simulink model "DAS"  (R2012b)
settings: Solver=FixedStepDiscrete  StartTime=0.0  StopTime=inf  FixedStep=0.1  RelTol=1e-3
PreLoadFcn:
  | if exist('tl_preloadfcn','file'), tl_preloadfcn(gcs,101); end
PostLoadFcn:
  | if exist('tl_postloadfcn','file'), tl_postloadfcn(gcs,101); end
InitFcn:
  | if exist('tlds_init','file'), tlds_init(gcs); end
StartFcn:
  | if exist('tlds_start','file'), tlds_start(gcs); end
StopFcn:
  | if exist('tlds_stop','file'), tlds_stop(gcs); end
undefined symbols (not defined in the file): A, B, C, Dd, DEMO_FAS_Accusti_Threshold_Time, DEMO_FAS_BrakeBooster_Threshold, DEMO_FAS_CC_DELTA, DEMO_FAS_CC_Lvl2_Round, DEMO_FAS_CC_Min_Value, DEMO_FAS_Distance_Treshold_Far, DEMO_FAS_Distance_Treshold_Med, DEMO_FAS_Distance_Treshold_Near, DEMO_FAS_Distronic, DEMO_FAS_Emerg_Brake_Force1, DEMO_FAS_Emerg_Brake_Force2, DEMO_FAS_Emerg_Brake_Time1, DEMO_FAS_Emerg_Brake_Time2, DEMO_FAS_EmergencyBrake, DEMO_FAS_FollowToStop, DEMO_FAS_Limiter, DEMO_FAS_Limiter_DELTA, DEMO_FAS_Neg_Max_ms, DEMO_FAS_Opti_Threshold_Time, DEMO_FAS_Repeater, DEMO_FAS_Repeater_Time, DEMO_FAS_Signdetection, DEMO_FAS_Tempomat
(part 8 of 11)

== system DAS/DEMO_FAS/DEMO_FAS/Subsystem/DEMO_FAS/DEMO_FAS_Funktion/Tempomat/Tempomat_Function/CC_Enabled/Tempomat_Active ==
  V_Vehicle_kmh : Inport
  Action Port : ActionPort  ActionType=then
  Data Store Read1 : DataStoreRead  Description=|  DataStoreName=DEMO_FAS_V_CCSetValue  mask(TL_DataStoreRead){data={'logdata',{'plotchannels',[]},'date',735342.58789737266}}
      | Data Store Read block of dSPACE TargetLink.
      | Use this block to specify inputs from global variables within the production code application.
      settings: DeleteFcn=if exist('delete_tlblock','file')==2,delete_tlblock(gcbh);end  NameChangeFcn=if exist('rename_tlblock','file')==2,rename_tlblock(gcbh);end  OpenFcn=if exist('tl_open_blockdlg','file')==2,tl_open_blockdlg(gcbh);else,open_system(gcbh,'parameter');end
      mask Help: eval(['if exist(''tl_online_help'',''file'') == 2, tl_online_help(''Topic'',''TL_DataStoreRead''),else, web([''jar:file:///'',matlabroot,''/help/toolbox/simulink/help.jar!/slref/' lower(get_param(gcbh,'Blocktype')) '.html''], ''-helpbrowser''),end'])
      mask Display: plot([-0.05, 1.05, NaN, -0.05, 1.05],[.01, .01, NaN, .99, .99])
  Sum : Sum  Description=|  Inputs=-+  mask(TL_Sum){data={'logdata',{'plotchannels',[]},'date',735350.38399912033}}
      | Sum block of dSPACE TargetLink.
      | 
      | Output signal is equal to the sum of the input signals.
      | The list of signs is specified according to conventions for Simulink Sum blocks.
      settings: CopyFcn=if exist('tl_reset_reviewflag') == 2, tl_reset_reviewflag(gcbh); end  DeleteFcn=if exist('delete_tlblock','file')==2,delete_tlblock(gcbh);end  NameChangeFcn=if exist('rename_tlblock','file')==2,rename_tlblock(gcbh);end  OpenFcn=if exist('tl_open_blockdlg','file')==2,tl_open_blockdlg(gcbh);else,open_system(gcbh,'parameter');end
      mask Help: eval(['if exist(''tl_online_help'',''file'') == 2, tl_online_help(''Topic'',''TL_Sum''),else, web([''jar:file:///'',matlabroot,''/help/toolbox/simulink/help.jar!/slref/' lower(get_param(gcbh,'Blocktype')) '.html''], ''-helpbrowser''),end'])
      mask Display: plot([-0.05, 1.05, NaN, -0.05, 1.05],[.01, .01, NaN, .99, .99])
  VERSION_INFO : Subsystem  mask(VERSION_INFO_BLOCK){versinfo_data=struct('modname','DEMO_FAS/DEMO_FAS_Funktion/Tempomat/Tempomat_Function/CC_Enabled/Tempomat_Active','version','1.1.1','date','18-Apr-2013','author','YVEDUHR','modtype',3,'variant',0,'remark',{{'~'}},'copyright',['Daimler AG'],'SGMLdescr','','prefix','','pfx_act',0,'ntselect',3,'asize',0), versinfo_string=Model: DEMO_FAS/DEMO_FAS_Funktion/Tempomat/Tempomat_Function/CC_Enabled/Tempomat_Active\nVersion: 1.1.1\nDate: 18-Apr-2013\nAuthor: YVEDUHR\nModule: INTERNAL\n\nAll copyrights by Daimler AG}
      mask prompts: versinfo_data "Mask Parameter 1"; versinfo_string "Mask Parameter 2"
      mask help:
      | This is a Version Info Subsystem (empty)
      | All version Information is stored in Parameter "versinfo_data" and displayed
      settings: OpenFcn=edit_subsys_info('init')
      mask Display: disp(versinfo_string);
  V_CC_delta_kmh : Outport  InitialOutput=0
  wires:
  V_Vehicle_kmh/1 -> Sum/1
  Sum/1 -> V_CC_delta_kmh/1  "V_CC_delta_kmh"
  Data Store Read1/1 -> Sum/2

== system DAS/DEMO_FAS/DEMO_FAS/Subsystem/DEMO_FAS/DEMO_FAS_Funktion/Tempomat/Tempomat_Function/CC_Enabled/Tempomat_Deactive ==
  Action Port : ActionPort  ActionType=else
  Constant : Constant  Value=0  mask(TL_Constant){data={'date',735339.6780933796}}
      settings: CopyFcn=if exist('tl_reset_reviewflag') == 2, tl_reset_reviewflag(gcbh); end  DeleteFcn=if exist('delete_tlblock','file')==2,delete_tlblock(gcbh);end  NameChangeFcn=if exist('rename_tlblock','file')==2,rename_tlblock(gcbh);end  OpenFcn=if exist('tl_open_blockdlg','file')==2,tl_open_blockdlg(gcbh);else,open_system(gcbh,'parameter');end
      mask Help: eval(['if exist(''tl_online_help'',''file'') == 2, tl_online_help(''Topic'',''TL_Constant''),else, web([''jar:file:///'',matlabroot,''/help/toolbox/simulink/help.jar!/slref/' lower(get_param(gcbh,'Blocktype')) '.html''], ''-helpbrowser''),end'])
      mask Display: plot([-0.05, 1.05, NaN, -0.05, 1.05],[.01, .01, NaN, .99, .99])
  VERSION_INFO : Subsystem  mask(VERSION_INFO_BLOCK){versinfo_data=struct('modname','DEMO_FAS/DEMO_FAS_Funktion/Tempomat/Tempomat_Function/CC_Enabled/Tempomat_Deactive','version','1.1.1','date','18-Apr-2013','author','YVEDUHR','modtype',3,'variant',0,'remark',{{'~'}},'copyright',['Daimler AG'],'SGMLdescr','','prefix','','pfx_act',0,'ntselect',3,'asize',0), versinfo_string=Model: DEMO_FAS/DEMO_FAS_Funktion/Tempomat/Tempomat_Function/CC_Enabled/Tempomat_Deactive\nVersion: 1.1.1\nDate: 18-Apr-2013\nAuthor: YVEDUHR\nModule: INTERNAL\n\nAll copyrights by Daimler AG}
      mask prompts: versinfo_data "Mask Parameter 1"; versinfo_string "Mask Parameter 2"
      mask help:
      | This is a Version Info Subsystem (empty)
      | All version Information is stored in Parameter "versinfo_data" and displayed
      settings: OpenFcn=edit_subsys_info('init')
      mask Display: disp(versinfo_string);
  V_CC_delta_kmh : Outport  InitialOutput=0
  wires:
  Constant/1 -> V_CC_delta_kmh/1  "V_CC_delta_kmh"

== system DAS/DEMO_FAS/DEMO_FAS/Subsystem/DEMO_FAS/DEMO_FAS_Funktion/Tempomat/Tempomat_Function/CC_Enabled/VERSION_INFO ==
  Copyright : Subsystem
      mask help: Copyright
      mask Display: disp('All copyrights by DaimlerChrysler');

== system DAS/DEMO_FAS/DEMO_FAS/Subsystem/DEMO_FAS/DEMO_FAS_Funktion/Tempomat/Tempomat_Function/CC_On_Off/EdgeFalling ==
  u : Inport
  R : Inport  Port=2
  IV : Inport  Port=3
  LogOp_A : Logic  Description=|  AllPortsSameDT=off  mask(TL_LogicalOperator){data={'logdata',{'plotchannels',[]},'date',734383.73416718747}}
      | Logical operator block of dSPACE TargetLink.
      | 
      | The Logical Operator block performs any of these logical operations on its inputs: AND, OR, NAND, NOR, XOR, and NOT. A nonzero input is treated as TRUE (1), a zero input as FALSE (0). The output depends on the selected operator. The output is 1 if TRUE and 0 if FALSE.
      settings: DeleteFcn=if exist('delete_tlblock','file')==2,delete_tlblock(gcbh);end  NameChangeFcn=if exist('rename_tlblock','file')==2,rename_tlblock(gcbh);end  OpenFcn=if exist('tl_open_blockdlg','file')==2,tl_open_blockdlg(gcbh);else,open_system(gcbh,'parameter');end
      mask Help: eval(['if exist(''tl_online_help'',''file'') == 2, tl_online_help(''Topic'',''TL_LogicalOperator''),else, web([''jar:file:///'',matlabroot,''/help/toolbox/simulink/help.jar!/slref/' lower(get_param(gcbh,'Blocktype')) '.html''], ''-helpbrowser''),end'])
      mask Display: plot([-0.05, 1.05, NaN, -0.05, 1.05],[.01, .01, NaN, .99, .99])
  LogOp_N : Logic  Description=|  Operator=NOT  Inputs=1  AllPortsSameDT=off  mask(TL_LogicalOperator){data={'logdata',{'plotchannels',[]},'date',734383.73416682868}}
      | Logical operator block of dSPACE TargetLink.
      | 
      | The Logical Operator block performs any of these logical operations on its inputs: AND, OR, NAND, NOR, XOR, and NOT. A nonzero input is treated as TRUE (1), a zero input as FALSE (0). The output depends on the selected operator. The output is 1 if TRUE and 0 if FALSE.
      settings: DeleteFcn=if exist('delete_tlblock','file')==2,delete_tlblock(gcbh);end  NameChangeFcn=if exist('rename_tlblock','file')==2,rename_tlblock(gcbh);end  OpenFcn=if exist('tl_open_blockdlg','file')==2,tl_open_blockdlg(gcbh);else,open_system(gcbh,'parameter');end
      mask Help: eval(['if exist(''tl_online_help'',''file'') == 2, tl_online_help(''Topic'',''TL_LogicalOperator''),else, web([''jar:file:///'',matlabroot,''/help/toolbox/simulink/help.jar!/slref/' lower(get_param(gcbh,'Blocktype')) '.html''], ''-helpbrowser''),end'])
      mask Display: plot([-0.05, 1.05, NaN, -0.05, 1.05],[.01, .01, NaN, .99, .99])
  Memory_U : UnitDelay  Description=|  SampleTime=dT  mask(TL_UnitDelay){data={'logdata',{'plotchannels',[]},'output',{'type','Bool'},'state',{'type','Bool'},'date',734383.73416645837}}
      | Unit Delay block of dSPACE TargetLink.
      | 
      | Output signal is equal to the input signal of the last sample step:
      | 
      |         y(k) = u(k-1).
      | 
      | In the 1st sampling step, the output signal is initialized with 'initial condition':
      | 
      |         y(0) = initial condition
      settings: CopyFcn=if exist('tl_reset_reviewflag') == 2, tl_reset_reviewflag(gcbh); end  DeleteFcn=if exist('delete_tlblock','file')==2,delete_tlblock(gcbh);end  NameChangeFcn=if exist('rename_tlblock','file')==2,rename_tlblock(gcbh);end  OpenFcn=if exist('tl_open_blockdlg','file')==2,tl_open_blockdlg(gcbh);else,open_system(gcbh,'parameter');end
      mask Help: eval(['if exist(''tl_online_help'',''file'') == 2, tl_online_help(''Topic'',''TL_UnitDelay''),else, web([''jar:file:///'',matlabroot,''/help/toolbox/simulink/help.jar!/slref/' lower(get_param(gcbh,'Blocktype')) '.html''], ''-helpbrowser''),end'])
      mask Display: plot([-0.05, 1.05, NaN, -0.05, 1.05],[.01, .01, NaN, .99, .99])
  Switch_R : Switch  Description=|  Threshold=1  mask(TL_Switch){data={'logdata',{'plotchannels',[]},'output',{'type','Bool'},'date',734383.73416555556}}
      | Switch block of dSPACE TargetLink.
      | 
      | Passes through input 1 if input 2 is greater than or equal to threshold, otherwise, passes through input 3:
      | 
      | if u2 >= threshold
      |    y = u1;
      | else
      |    y = u3;
      | end
      settings: CopyFcn=if exist('tl_reset_reviewflag') == 2, tl_reset_reviewflag(gcbh); end  DeleteFcn=if exist('delete_tlblock','file')==2,delete_tlblock(gcbh);end  NameChangeFcn=if exist('rename_tlblock','file')==2,rename_tlblock(gcbh);end  OpenFcn=if exist('tl_open_blockdlg','file')==2,tl_open_blockdlg(gcbh);else,open_system(gcbh,'parameter');end
      mask Help: eval(['if exist(''tl_online_help'',''file'') == 2, tl_online_help(''Topic'',''TL_Switch''),else, web([''jar:file:///'',matlabroot,''/help/toolbox/simulink/help.jar!/slref/' lower(get_param(gcbh,'Blocktype')) '.html''], ''-helpbrowser''),end'])
      mask Display: plot([-0.05, 1.05, NaN, -0.05, 1.05],[.01, .01, NaN, .99, .99])
  y : Outport  InitialOutput=0
  wires:
  IV/1 -> Switch_R/1
  Memory_U/1 -> Switch_R/3
  R/1 -> Switch_R/2
  LogOp_A/1 -> y/1
  LogOp_N/1 -> LogOp_A/1
  u/1 -> Memory_U/1, LogOp_N/1
  Switch_R/1 -> LogOp_A/2

== system DAS/DEMO_FAS/DEMO_FAS/Subsystem/DEMO_FAS/DEMO_FAS_Funktion/Tempomat/Tempomat_Function/CC_On_Off/EdgeRising1 ==
  u : Inport
  R : Inport  Port=2
  IV : Inport  Port=3
  LogOp_A : Logic  Description=|  AllPortsSameDT=off  mask(TL_LogicalOperator){data={'logdata',{'plotchannels',[]},'date',734383.73416157404}}
      | Logical operator block of dSPACE TargetLink.
      | 
      | The Logical Operator block performs any of these logical operations on its inputs: AND, OR, NAND, NOR, XOR, and NOT. A nonzero input is treated as TRUE (1), a zero input as FALSE (0). The output depends on the selected operator. The output is 1 if TRUE and 0 if FALSE.
      settings: DeleteFcn=if exist('delete_tlblock','file')==2,delete_tlblock(gcbh);end  NameChangeFcn=if exist('rename_tlblock','file')==2,rename_tlblock(gcbh);end  OpenFcn=if exist('tl_open_blockdlg','file')==2,tl_open_blockdlg(gcbh);else,open_system(gcbh,'parameter');end
      mask Help: eval(['if exist(''tl_online_help'',''file'') == 2, tl_online_help(''Topic'',''TL_LogicalOperator''),else, web([''jar:file:///'',matlabroot,''/help/toolbox/simulink/help.jar!/slref/' lower(get_param(gcbh,'Blocktype')) '.html''], ''-helpbrowser''),end'])
      mask Display: plot([-0.05, 1.05, NaN, -0.05, 1.05],[.01, .01, NaN, .99, .99])
  LogOp_N : Logic  Description=|  Operator=NOT  Inputs=1  AllPortsSameDT=off  mask(TL_LogicalOperator){data={'logdata',{'plotchannels',[]},'date',734383.73416121525}}
      | Logical operator block of dSPACE TargetLink.
      | 
      | The Logical Operator block performs any of these logical operations on its inputs: AND, OR, NAND, NOR, XOR, and NOT. A nonzero input is treated as TRUE (1), a zero input as FALSE (0). The output depends on the selected operator. The output is 1 if TRUE and 0 if FALSE.
      settings: DeleteFcn=if exist('delete_tlblock','file')==2,delete_tlblock(gcbh);end  NameChangeFcn=if exist('rename_tlblock','file')==2,rename_tlblock(gcbh);end  OpenFcn=if exist('tl_open_blockdlg','file')==2,tl_open_blockdlg(gcbh);else,open_system(gcbh,'parameter');end
      mask Help: eval(['if exist(''tl_online_help'',''file'') == 2, tl_online_help(''Topic'',''TL_LogicalOperator''),else, web([''jar:file:///'',matlabroot,''/help/toolbox/simulink/help.jar!/slref/' lower(get_param(gcbh,'Blocktype')) '.html''], ''-helpbrowser''),end'])
      mask Display: plot([-0.05, 1.05, NaN, -0.05, 1.05],[.01, .01, NaN, .99, .99])
  Memory_U : UnitDelay  Description=|  SampleTime=dT  mask(TL_UnitDelay){data={'logdata',{'plotchannels',[]},'output',{'type','Bool'},'state',{'type','Bool'},'date',734383.73416067124}}
      | Unit Delay block of dSPACE TargetLink.
      | 
      | Output signal is equal to the input signal of the last sample step:
      | 
      |         y(k) = u(k-1).
      | 
      | In the 1st sampling step, the output signal is initialized with 'initial condition':
      | 
      |         y(0) = initial condition
      settings: CopyFcn=if exist('tl_reset_reviewflag') == 2, tl_reset_reviewflag(gcbh); end  DeleteFcn=if exist('delete_tlblock','file')==2,delete_tlblock(gcbh);end  NameChangeFcn=if exist('rename_tlblock','file')==2,rename_tlblock(gcbh);end  OpenFcn=if exist('tl_open_blockdlg','file')==2,tl_open_blockdlg(gcbh);else,open_system(gcbh,'parameter');end
      mask Help: eval(['if exist(''tl_online_help'',''file'') == 2, tl_online_help(''Topic'',''TL_UnitDelay''),else, web([''jar:file:///'',matlabroot,''/help/toolbox/simulink/help.jar!/slref/' lower(get_param(gcbh,'Blocktype')) '.html''], ''-helpbrowser''),end'])
      mask Display: plot([-0.05, 1.05, NaN, -0.05, 1.05],[.01, .01, NaN, .99, .99])
  Switch_R : Switch  Description=|  Threshold=1  mask(TL_Switch){data={'logdata',{'plotchannels',[]},'output',{'type','Bool'},'date',734383.73415995366}}
      | Switch block of dSPACE TargetLink.
      | 
      | Passes through input 1 if input 2 is greater than or equal to threshold, otherwise, passes through input 3:
      | 
      | if u2 >= threshold
      |    y = u1;
      | else
      |    y = u3;
      | end
      settings: CopyFcn=if exist('tl_reset_reviewflag') == 2, tl_reset_reviewflag(gcbh); end  DeleteFcn=if exist('delete_tlblock','file')==2,delete_tlblock(gcbh);end  NameChangeFcn=if exist('rename_tlblock','file')==2,rename_tlblock(gcbh);end  OpenFcn=if exist('tl_open_blockdlg','file')==2,tl_open_blockdlg(gcbh);else,open_system(gcbh,'parameter');end
      mask Help: eval(['if exist(''tl_online_help'',''file'') == 2, tl_online_help(''Topic'',''TL_Switch''),else, web([''jar:file:///'',matlabroot,''/help/toolbox/simulink/help.jar!/slref/' lower(get_param(gcbh,'Blocktype')) '.html''], ''-helpbrowser''),end'])
      mask Display: plot([-0.05, 1.05, NaN, -0.05, 1.05],[.01, .01, NaN, .99, .99])
  y : Outport  InitialOutput=0
  wires:
  LogOp_N/1 -> LogOp_A/2
  LogOp_A/1 -> y/1
  u/1 -> LogOp_A/1, Memory_U/1
  Switch_R/1 -> LogOp_N/1
  R/1 -> Switch_R/2
  Memory_U/1 -> Switch_R/3
  IV/1 -> Switch_R/1

== system DAS/DEMO_FAS/DEMO_FAS/Subsystem/DEMO_FAS/DEMO_FAS_Funktion/Tempomat/Tempomat_Function/CC_On_Off/False1 ==
  Zero : Constant  Description=|  Value=0  SampleTime=-1  mask(TL_Constant){data={'output',{'tolerance',0},'date',734383.73403155094}}
      | Constant block of dSPACE TargetLink.
      | 
      | Output signal keeps the given constant value.
      settings: DeleteFcn=if exist('delete_tlblock','file')==2,delete_tlblock(gcbh);end  NameChangeFcn=if exist('rename_tlblock','file')==2,rename_tlblock(gcbh);end  OpenFcn=if exist('tl_open_blockdlg','file')==2,tl_open_blockdlg(gcbh);else,open_system(gcbh,'parameter');end
      mask Help: eval(['if exist(''tl_online_help'',''file'') == 2, tl_online_help(''Topic'',''TL_Constant''),else, web([''jar:file:///'',matlabroot,''/help/toolbox/simulink/help.jar!/slref/' lower(get_param(gcbh,'Blocktype')) '.html''], ''-helpbrowser''),end'])
      mask Display: plot([-0.05, 1.05, NaN, -0.05, 1.05],[.01, .01, NaN, .99, .99])
  y : Outport
  wires:
  Zero/1 -> y/1

== system DAS/DEMO_FAS/DEMO_FAS/Subsystem/DEMO_FAS/DEMO_FAS_Funktion/Tempomat/Tempomat_Function/CC_On_Off/False2 ==
  Zero : Constant  Description=|  Value=0  SampleTime=-1  mask(TL_Constant){data={'output',{'tolerance',0},'date',734383.73403155094}}
      | Constant block of dSPACE TargetLink.
      | 
      | Output signal keeps the given constant value.
      settings: DeleteFcn=if exist('delete_tlblock','file')==2,delete_tlblock(gcbh);end  NameChangeFcn=if exist('rename_tlblock','file')==2,rename_tlblock(gcbh);end  OpenFcn=if exist('tl_open_blockdlg','file')==2,tl_open_blockdlg(gcbh);else,open_system(gcbh,'parameter');end
      mask Help: eval(['if exist(''tl_online_help'',''file'') == 2, tl_online_help(''Topic'',''TL_Constant''),else, web([''jar:file:///'',matlabroot,''/help/toolbox/simulink/help.jar!/slref/' lower(get_param(gcbh,'Blocktype')) '.html''], ''-helpbrowser''),end'])
      mask Display: plot([-0.05, 1.05, NaN, -0.05, 1.05],[.01, .01, NaN, .99, .99])
  y : Outport
  wires:
  Zero/1 -> y/1

== system DAS/DEMO_FAS/DEMO_FAS/Subsystem/DEMO_FAS/DEMO_FAS_Funktion/Tempomat/Tempomat_Function/CC_On_Off/RSFlipFlop ==
  S : Inport
  R : Inport  Port=2
  LogOp_N : Logic  Description=|  Operator=NOT  Inputs=1  AllPortsSameDT=off  mask(TL_LogicalOperator){data={'logdata',{'plotchannels',[]},'date',734383.73415922455}}
      | Logical operator block of dSPACE TargetLink.
      | 
      | The Logical Operator block performs any of these logical operations on its inputs: AND, OR, NAND, NOR, XOR, and NOT. A nonzero input is treated as TRUE (1), a zero input as FALSE (0). The output depends on the selected operator. The output is 1 if TRUE and 0 if FALSE.
      settings: DeleteFcn=if exist('delete_tlblock','file')==2,delete_tlblock(gcbh);end  NameChangeFcn=if exist('rename_tlblock','file')==2,rename_tlblock(gcbh);end  OpenFcn=if exist('tl_open_blockdlg','file')==2,tl_open_blockdlg(gcbh);else,open_system(gcbh,'parameter');end
      mask Help: eval(['if exist(''tl_online_help'',''file'') == 2, tl_online_help(''Topic'',''TL_LogicalOperator''),else, web([''jar:file:///'',matlabroot,''/help/toolbox/simulink/help.jar!/slref/' lower(get_param(gcbh,'Blocktype')) '.html''], ''-helpbrowser''),end'])
      mask Display: plot([-0.05, 1.05, NaN, -0.05, 1.05],[.01, .01, NaN, .99, .99])
  Memory_Q : UnitDelay  Description=|  SampleTime=dT  mask(TL_UnitDelay){data={'logdata',{'plotchannels',[]},'output',{'type','Bool'},'state',{'type','Bool'},'date',734383.73415886576}}
      | Unit Delay block of dSPACE TargetLink.
      | 
      | Output signal is equal to the input signal of the last sample step:
      | 
      |         y(k) = u(k-1).
      | 
      | In the 1st sampling step, the output signal is initialized with 'initial condition':
      | 
      |         y(0) = initial condition
      settings: CopyFcn=if exist('tl_reset_reviewflag') == 2, tl_reset_reviewflag(gcbh); end  DeleteFcn=if exist('delete_tlblock','file')==2,delete_tlblock(gcbh);end  NameChangeFcn=if exist('rename_tlblock','file')==2,rename_tlblock(gcbh);end  OpenFcn=if exist('tl_open_blockdlg','file')==2,tl_open_blockdlg(gcbh);else,open_system(gcbh,'parameter');end
      mask Help: eval(['if exist(''tl_online_help'',''file'') == 2, tl_online_help(''Topic'',''TL_UnitDelay''),else, web([''jar:file:///'',matlabroot,''/help/toolbox/simulink/help.jar!/slref/' lower(get_param(gcbh,'Blocktype')) '.html''], ''-helpbrowser''),end'])
      mask Display: plot([-0.05, 1.05, NaN, -0.05, 1.05],[.01, .01, NaN, .99, .99])
  One_S : Constant  Description=|  mask(TL_Constant){data={'date',734383.73415796296}}
      | Constant block of dSPACE TargetLink.
      | 
      | Output signal keeps the given constant value.
      settings: DeleteFcn=if exist('delete_tlblock','file')==2,delete_tlblock(gcbh);end  NameChangeFcn=if exist('rename_tlblock','file')==2,rename_tlblock(gcbh);end  OpenFcn=if exist('tl_open_blockdlg','file')==2,tl_open_blockdlg(gcbh);else,open_system(gcbh,'parameter');end
      mask Help: eval(['if exist(''tl_online_help'',''file'') == 2, tl_online_help(''Topic'',''TL_Constant''),else, web([''jar:file:///'',matlabroot,''/help/toolbox/simulink/help.jar!/slref/' lower(get_param(gcbh,'Blocktype')) '.html''], ''-helpbrowser''),end'])
      mask Display: plot([-0.05, 1.05, NaN, -0.05, 1.05],[.01, .01, NaN, .99, .99])
  Switch_R : Switch  Description=|  Threshold=1  mask(TL_Switch){data={'logdata',{'plotchannels',[]},'output',{'type','Bool'},'date',734383.73415760417}}
      | Switch block of dSPACE TargetLink.
      | 
      | Passes through input 1 if input 2 is greater than or equal to threshold, otherwise, passes through input 3:
      | 
      | if u2 >= threshold
      |    y = u1;
      | else
      |    y = u3;
      | end
      settings: CopyFcn=if exist('tl_reset_reviewflag') == 2, tl_reset_reviewflag(gcbh); end  DeleteFcn=if exist('delete_tlblock','file')==2,delete_tlblock(gcbh);end  NameChangeFcn=if exist('rename_tlblock','file')==2,rename_tlblock(gcbh);end  OpenFcn=if exist('tl_open_blockdlg','file')==2,tl_open_blockdlg(gcbh);else,open_system(gcbh,'parameter');end
      mask Help: eval(['if exist(''tl_online_help'',''file'') == 2, tl_online_help(''Topic'',''TL_Switch''),else, web([''jar:file:///'',matlabroot,''/help/toolbox/simulink/help.jar!/slref/' lower(get_param(gcbh,'Blocktype')) '.html''], ''-helpbrowser''),end'])
      mask Display: plot([-0.05, 1.05, NaN, -0.05, 1.05],[.01, .01, NaN, .99, .99])
  Switch_S : Switch  Description=|  Threshold=1  mask(TL_Switch){data={'logdata',{'plotchannels',[]},'output',{'type','Bool'},'date',734383.73415668984}}
      | Switch block of dSPACE TargetLink.
      | 
      | Passes through input 1 if input 2 is greater than or equal to threshold, otherwise, passes through input 3:
      | 
      | if u2 >= threshold
      |    y = u1;
      | else
      |    y = u3;
      | end
      settings: CopyFcn=if exist('tl_reset_reviewflag') == 2, tl_reset_reviewflag(gcbh); end  DeleteFcn=if exist('delete_tlblock','file')==2,delete_tlblock(gcbh);end  NameChangeFcn=if exist('rename_tlblock','file')==2,rename_tlblock(gcbh);end  OpenFcn=if exist('tl_open_blockdlg','file')==2,tl_open_blockdlg(gcbh);else,open_system(gcbh,'parameter');end
      mask Help: eval(['if exist(''tl_online_help'',''file'') == 2, tl_online_help(''Topic'',''TL_Switch''),else, web([''jar:file:///'',matlabroot,''/help/toolbox/simulink/help.jar!/slref/' lower(get_param(gcbh,'Blocktype')) '.html''], ''-helpbrowser''),end'])
      mask Display: plot([-0.05, 1.05, NaN, -0.05, 1.05],[.01, .01, NaN, .99, .99])
  Zero_R : Constant  Description=|  Value=0  mask(TL_Constant){data={'date',734383.73415597226}}
      | Constant block of dSPACE TargetLink.
      | 
      | Output signal keeps the given constant value.
      settings: DeleteFcn=if exist('delete_tlblock','file')==2,delete_tlblock(gcbh);end  NameChangeFcn=if exist('rename_tlblock','file')==2,rename_tlblock(gcbh);end  OpenFcn=if exist('tl_open_blockdlg','file')==2,tl_open_blockdlg(gcbh);else,open_system(gcbh,'parameter');end
      mask Help: eval(['if exist(''tl_online_help'',''file'') == 2, tl_online_help(''Topic'',''TL_Constant''),else, web([''jar:file:///'',matlabroot,''/help/toolbox/simulink/help.jar!/slref/' lower(get_param(gcbh,'Blocktype')) '.html''], ''-helpbrowser''),end'])
      mask Display: plot([-0.05, 1.05, NaN, -0.05, 1.05],[.01, .01, NaN, .99, .99])
  Q : Outport  InitialOutput=0
  NOT_Q : Outport  Port=2  InitialOutput=0
  wires:
  LogOp_N/1 -> NOT_Q/1
  R/1 -> Switch_R/2
  Zero_R/1 -> Switch_R/1
  Switch_R/1 -> LogOp_N/1, Q/1, Memory_Q/1
  S/1 -> Switch_S/2
  One_S/1 -> Switch_S/1
  Switch_S/1 -> Switch_R/3
  Memory_Q/1 -> Switch_S/3

== system DAS/DEMO_FAS/DEMO_FAS/Subsystem/DEMO_FAS/DEMO_FAS_Funktion/Tempomat/Tempomat_Function/CC_On_Off/VERSION_INFO ==
  Copyright : Subsystem
      mask help: Copyright
      mask Display: disp('All copyrights by DaimlerChrysler');

== system DAS/DEMO_FAS/DEMO_FAS/Subsystem/DEMO_FAS/DEMO_FAS_Funktion/Tempomat/Tempomat_Function/CC_SetValue/CC_ChangeSetValue ==
  LeverUp_stat : Inport
  LeverDown_stat : Inport  Port=2
  Enable : EnablePort
  CC_ChangeSetValue_Lvl2_Repeater : Subsystem
  CC_ChangeSetValue_Lvl2_no_Repeater : Subsystem
  DEMO_FAS_Repeater : Constant  Description=|  Value=DEMO_FAS_Repeater  SampleTime=-1  mask(TL_Constant){data={'output',{'variable','DEMO_FAS/p/Components/DEMO_FAS_Repeater'},'date',735354.40861667821}}
      | Constant block of dSPACE TargetLink.
      | 
      | Output signal keeps the given constant value.
      settings: DeleteFcn=if exist('delete_tlblock','file')==2,delete_tlblock(gcbh);end  NameChangeFcn=if exist('rename_tlblock','file')==2,rename_tlblock(gcbh);end  OpenFcn=if exist('tl_open_blockdlg','file')==2,tl_open_blockdlg(gcbh);else,open_system(gcbh,'parameter');end
      mask Help: eval(['if exist(''tl_online_help'',''file'') == 2, tl_online_help(''Topic'',''TL_Constant''),else, web([''jar:file:///'',matlabroot,''/help/toolbox/simulink/help.jar!/slref/' lower(get_param(gcbh,'Blocktype')) '.html''], ''-helpbrowser''),end'])
      mask Display: plot([-0.05, 1.05, NaN, -0.05, 1.05],[.01, .01, NaN, .99, .99])
  If : If  IfExpression=~u1  ElseIfExpressions=u1  ShowElse=off
  VERSION_INFO : Subsystem  mask(VERSION_INFO_BLOCK){versinfo_data=struct('modname','DEMO_FAS/DEMO_FAS_Funktion/Tempomat/Tempomat_Function/CC_SetValue/CC_ChangeSetValue','version','1.1.1','date','22-Apr-2013','author','YVEDUHR','modtype',3,'variant',0,'remark',{{'~'}},'copyright',['Daimler AG'],'SGMLdescr','','prefix','','pfx_act',0,'ntselect',3,'asize',0), versinfo_string=Model: DEMO_FAS/DEMO_FAS_Funktion/Tempomat/Tempomat_Function/CC_SetValue/CC_ChangeSetValue\nVersion: 1.1.1\nDate: 22-Apr-2013\nAuthor: YVEDUHR\nModule: INTERNAL\n\nAll copyrights by Daimler AG}
      mask prompts: versinfo_data "Mask Parameter 1"; versinfo_string "Mask Parameter 2"
      mask help:
      | This is a Version Info Subsystem (empty)
      | All version Information is stored in Parameter "versinfo_data" and displayed
      settings: OpenFcn=edit_subsys_info('init')
      mask Display: disp(versinfo_string);
  wires:
  LeverUp_stat/1 -> CC_ChangeSetValue_Lvl2_Repeater/1(LeverUp_Stat), CC_ChangeSetValue_Lvl2_no_Repeater/1(LeverUp_stat)
  DEMO_FAS_Repeater/1 -> If/1
  LeverDown_stat/1 -> CC_ChangeSetValue_Lvl2_Repeater/2(LeverDown_Stat), CC_ChangeSetValue_Lvl2_no_Repeater/2(LeverDown_stat)
  If/1 -> CC_ChangeSetValue_Lvl2_no_Repeater/Action
  If/2 -> CC_ChangeSetValue_Lvl2_Repeater/Action

== system DAS/DEMO_FAS/DEMO_FAS/Subsystem/DEMO_FAS/DEMO_FAS_Funktion/Tempomat/Tempomat_Function/CC_SetValue/CC_InitialSetValue ==
  V_Vehicle_kmh : Inport
  Trigger : TriggerPort
  CC_NoInitialSetValue : Subsystem  TreatAsAtomicUnit=on
  Constant : Constant  Value=0  mask(TL_Constant){data={'date',735343.64483707177}}
      settings: CopyFcn=if exist('tl_reset_reviewflag') == 2, tl_reset_reviewflag(gcbh); end  DeleteFcn=if exist('delete_tlblock','file')==2,delete_tlblock(gcbh);end  NameChangeFcn=if exist('rename_tlblock','file')==2,rename_tlblock(gcbh);end  OpenFcn=if exist('tl_open_blockdlg','file')==2,tl_open_blockdlg(gcbh);else,open_system(gcbh,'parameter');end
      mask Help: eval(['if exist(''tl_online_help'',''file'') == 2, tl_online_help(''Topic'',''TL_Constant''),else, web([''jar:file:///'',matlabroot,''/help/toolbox/simulink/help.jar!/slref/' lower(get_param(gcbh,'Blocktype')) '.html''], ''-helpbrowser''),end'])
      mask Display: plot([-0.05, 1.05, NaN, -0.05, 1.05],[.01, .01, NaN, .99, .99])
  Data Store Read1 : DataStoreRead  Description=|  DataStoreName=DEMO_FAS_V_CCSetValue  mask(TL_DataStoreRead){data={'logdata',{'plotchannels',[]},'date',735342.58789737266}}
      | Data Store Read block of dSPACE TargetLink.
      | Use this block to specify inputs from global variables within the production code application.
      settings: DeleteFcn=if exist('delete_tlblock','file')==2,delete_tlblock(gcbh);end  NameChangeFcn=if exist('rename_tlblock','file')==2,rename_tlblock(gcbh);end  OpenFcn=if exist('tl_open_blockdlg','file')==2,tl_open_blockdlg(gcbh);else,open_system(gcbh,'parameter');end
      mask Help: eval(['if exist(''tl_online_help'',''file'') == 2, tl_online_help(''Topic'',''TL_DataStoreRead''),else, web([''jar:file:///'',matlabroot,''/help/toolbox/simulink/help.jar!/slref/' lower(get_param(gcbh,'Blocktype')) '.html''], ''-helpbrowser''),end'])
      mask Display: plot([-0.05, 1.05, NaN, -0.05, 1.05],[.01, .01, NaN, .99, .99])
  If : If  IfExpression=u1  ShowElse=off
  RelOp : RelationalOperator  Description=|  Operator=<  mask(TL_RelationalOperator){data={'logdata',{'plotchannels',[]},'date',735343.64478756941}}
      | Relational operator block of dSPACE TargetLink.
      | 
      | This block performs a relational operation on its two inputs u1 and u2 and produces output according to the following table.
      | If the result is TRUE, the output is 1; if FALSE, it is 0.
      | 
      | Operator   Output
      |  ==        TRUE if u1 is equal to u2
      |  !=        TRUE if u1 is not equal to u2
      |  <         TRUE if u1 is less than u2
      |  <=        TRUE if u1 is less than or equal to u2
      |  >=        TRUE if u1 is greater than or equal to u2
      |  >         TRUE if u1 is greater than u2
      settings: DeleteFcn=if exist('delete_tlblock','file')==2,delete_tlblock(gcbh);end  NameChangeFcn=if exist('rename_tlblock','file')==2,rename_tlblock(gcbh);end  OpenFcn=if exist('tl_open_blockdlg','file')==2,tl_open_blockdlg(gcbh);else,open_system(gcbh,'parameter');end
      mask Help: eval(['if exist(''tl_online_help'',''file'') == 2, tl_online_help(''Topic'',''TL_RelationalOperator''),else, web([''jar:file:///'',matlabroot,''/help/toolbox/simulink/help.jar!/slref/' lower(get_param(gcbh,'Blocktype')) '.html''], ''-helpbrowser''),end'])
      mask Display: plot([-0.05, 1.05, NaN, -0.05, 1.05],[.01, .01, NaN, .99, .99])
  VERSION_INFO : Subsystem  mask(VERSION_INFO_BLOCK){versinfo_data=struct('modname','DEMO_FAS/DEMO_FAS_Funktion/Tempomat/Tempomat_Function/CC_SetValue/CC_InitialSetValue','version','1.1.1','date','22-Apr-2013','author','YVEDUHR','modtype',3,'variant',0,'remark',{{'~'}},'copyright',['Daimler AG'],'SGMLdescr','','prefix','','pfx_act',0,'ntselect',3,'asize',0), versinfo_string=Model: DEMO_FAS/DEMO_FAS_Funktion/Tempomat/Tempomat_Function/CC_SetValue/CC_InitialSetValue\nVersion: 1.1.1\nDate: 22-Apr-2013\nAuthor: YVEDUHR\nModule: INTERNAL\n\nAll copyrights by Daimler AG}
      mask prompts: versinfo_data "Mask Parameter 1"; versinfo_string "Mask Parameter 2"
      mask help:
      | This is a Version Info Subsystem (empty)
      | All version Information is stored in Parameter "versinfo_data" and displayed
      settings: OpenFcn=edit_subsys_info('init')
      mask Display: disp(versinfo_string);
  wires:
  V_Vehicle_kmh/1 -> CC_NoInitialSetValue/1(V_Vehicle_kmh)
  Constant/1 -> RelOp/2
  Data Store Read1/1 -> RelOp/1
  RelOp/1 -> If/1
  If/1 -> CC_NoInitialSetValue/Action

== system DAS/DEMO_FAS/DEMO_FAS/Subsystem/DEMO_FAS/DEMO_FAS_Funktion/Tempomat/Tempomat_Function/CC_SetValue/CC_OnSet_SetValue ==
  V_Vehicle_kmh : Inport
  Trigger : TriggerPort
  Data Store Write : DataStoreWrite  Description=|  DataStoreName=DEMO_FAS_V_CCSetValue  mask(TL_DataStoreWrite){data={'date',735342.52876391204}}
      | Data Store Write block of dSPACE TargetLink.
      | Use this block to specify outputs to global variables within the production code application.
      settings: DeleteFcn=if exist('delete_tlblock','file')==2,delete_tlblock(gcbh);end  NameChangeFcn=if exist('rename_tlblock','file')==2,rename_tlblock(gcbh);end  OpenFcn=if exist('tl_open_blockdlg','file')==2,tl_open_blockdlg(gcbh);else,open_system(gcbh,'parameter');end
      mask Help: eval(['if exist(''tl_online_help'',''file'') == 2, tl_online_help(''Topic'',''TL_DataStoreWrite''),else, web([''jar:file:///'',matlabroot,''/help/toolbox/simulink/help.jar!/slref/' lower(get_param(gcbh,'Blocktype')) '.html''], ''-helpbrowser''),end'])
      mask Display: plot([-0.05, 1.05, NaN, -0.05, 1.05],[.01, .01, NaN, .99, .99])
  VERSION_INFO : Subsystem  mask(VERSION_INFO_BLOCK){versinfo_data=struct('modname','DEMO_FAS/DEMO_FAS_Funktion/Tempomat/Tempomat_Function/CC_SetValue/CC_OnSet_SetValue','version','1.1.1','date','22-Apr-2013','author','YVEDUHR','modtype',3,'variant',0,'remark',{{'~'}},'copyright',['Daimler AG'],'SGMLdescr','','prefix','','pfx_act',0,'ntselect',3,'asize',0), versinfo_string=Model: DEMO_FAS/DEMO_FAS_Funktion/Tempomat/Tempomat_Function/CC_SetValue/CC_OnSet_SetValue\nVersion: 1.1.1\nDate: 22-Apr-2013\nAuthor: YVEDUHR\nModule: INTERNAL\n\nAll copyrights by Daimler AG}
      mask prompts: versinfo_data "Mask Parameter 1"; versinfo_string "Mask Parameter 2"
      mask help:
      | This is a Version Info Subsystem (empty)
      | All version Information is stored in Parameter "versinfo_data" and displayed
      settings: OpenFcn=edit_subsys_info('init')
      mask Display: disp(versinfo_string);
  wires:
  V_Vehicle_kmh/1 -> Data Store Write/1

== system DAS/DEMO_FAS/DEMO_FAS/Subsystem/DEMO_FAS/DEMO_FAS_Funktion/Tempomat/Tempomat_Function/CC_SetValue/CC_StartUpSetValue ==
  Trigger : TriggerPort
  Constant : Constant  Value=-1  mask(TL_Constant){data={'date',735343.64397744217}}
      settings: CopyFcn=if exist('tl_reset_reviewflag') == 2, tl_reset_reviewflag(gcbh); end  DeleteFcn=if exist('delete_tlblock','file')==2,delete_tlblock(gcbh);end  NameChangeFcn=if exist('rename_tlblock','file')==2,rename_tlblock(gcbh);end  OpenFcn=if exist('tl_open_blockdlg','file')==2,tl_open_blockdlg(gcbh);else,open_system(gcbh,'parameter');end
      mask Help: eval(['if exist(''tl_online_help'',''file'') == 2, tl_online_help(''Topic'',''TL_Constant''),else, web([''jar:file:///'',matlabroot,''/help/toolbox/simulink/help.jar!/slref/' lower(get_param(gcbh,'Blocktype')) '.html''], ''-helpbrowser''),end'])
      mask Display: plot([-0.05, 1.05, NaN, -0.05, 1.05],[.01, .01, NaN, .99, .99])
  Data Store Write : DataStoreWrite  Description=|  DataStoreName=DEMO_FAS_V_CCSetValue  mask(TL_DataStoreWrite){data={'date',735342.52876391204}}
      | Data Store Write block of dSPACE TargetLink.
      | Use this block to specify outputs to global variables within the production code application.
      settings: DeleteFcn=if exist('delete_tlblock','file')==2,delete_tlblock(gcbh);end  NameChangeFcn=if exist('rename_tlblock','file')==2,rename_tlblock(gcbh);end  OpenFcn=if exist('tl_open_blockdlg','file')==2,tl_open_blockdlg(gcbh);else,open_system(gcbh,'parameter');end
      mask Help: eval(['if exist(''tl_online_help'',''file'') == 2, tl_online_help(''Topic'',''TL_DataStoreWrite''),else, web([''jar:file:///'',matlabroot,''/help/toolbox/simulink/help.jar!/slref/' lower(get_param(gcbh,'Blocktype')) '.html''], ''-helpbrowser''),end'])
      mask Display: plot([-0.05, 1.05, NaN, -0.05, 1.05],[.01, .01, NaN, .99, .99])
  VERSION_INFO : Subsystem  mask(VERSION_INFO_BLOCK){versinfo_data=struct('modname','DEMO_FAS/DEMO_FAS_Funktion/Tempomat/Tempomat_Function/CC_SetValue/CC_StartUpSetValue','version','1.1.1','date','22-Apr-2013','author','YVEDUHR','modtype',3,'variant',0,'remark',{{'~'}},'copyright',['Daimler AG'],'SGMLdescr','','prefix','','pfx_act',0,'ntselect',3,'asize',0), versinfo_string=Model: DEMO_FAS/DEMO_FAS_Funktion/Tempomat/Tempomat_Function/CC_SetValue/CC_StartUpSetValue\nVersion: 1.1.1\nDate: 22-Apr-2013\nAuthor: YVEDUHR\nModule: INTERNAL\n\nAll copyrights by Daimler AG}
      mask prompts: versinfo_data "Mask Parameter 1"; versinfo_string "Mask Parameter 2"
      mask help:
      | This is a Version Info Subsystem (empty)
      | All version Information is stored in Parameter "versinfo_data" and displayed
      settings: OpenFcn=edit_subsys_info('init')
      mask Display: disp(versinfo_string);
  wires:
  Constant/1 -> Data Store Write/1

== system DAS/DEMO_FAS/DEMO_FAS/Subsystem/DEMO_FAS/DEMO_FAS_Funktion/Tempomat/Tempomat_Function/CC_SetValue/EdgeRising ==
  u : Inport
  R : Inport  Port=2
  IV : Inport  Port=3
  LogOp_A : Logic  Description=|  AllPortsSameDT=off  mask(TL_LogicalOperator){data={'logdata',{'plotchannels',[]},'date',734383.73416157404}}
      | Logical operator block of dSPACE TargetLink.
      | 
      | The Logical Operator block performs any of these logical operations on its inputs: AND, OR, NAND, NOR, XOR, and NOT. A nonzero input is treated as TRUE (1), a zero input as FALSE (0). The output depends on the selected operator. The output is 1 if TRUE and 0 if FALSE.
      settings: DeleteFcn=if exist('delete_tlblock','file')==2,delete_tlblock(gcbh);end  NameChangeFcn=if exist('rename_tlblock','file')==2,rename_tlblock(gcbh);end  OpenFcn=if exist('tl_open_blockdlg','file')==2,tl_open_blockdlg(gcbh);else,open_system(gcbh,'parameter');end
      mask Help: eval(['if exist(''tl_online_help'',''file'') == 2, tl_online_help(''Topic'',''TL_LogicalOperator''),else, web([''jar:file:///'',matlabroot,''/help/toolbox/simulink/help.jar!/slref/' lower(get_param(gcbh,'Blocktype')) '.html''], ''-helpbrowser''),end'])
      mask Display: plot([-0.05, 1.05, NaN, -0.05, 1.05],[.01, .01, NaN, .99, .99])
  LogOp_N : Logic  Description=|  Operator=NOT  Inputs=1  AllPortsSameDT=off  mask(TL_LogicalOperator){data={'logdata',{'plotchannels',[]},'date',734383.73416121525}}
      | Logical operator block of dSPACE TargetLink.
      | 
      | The Logical Operator block performs any of these logical operations on its inputs: AND, OR, NAND, NOR, XOR, and NOT. A nonzero input is treated as TRUE (1), a zero input as FALSE (0). The output depends on the selected operator. The output is 1 if TRUE and 0 if FALSE.
      settings: DeleteFcn=if exist('delete_tlblock','file')==2,delete_tlblock(gcbh);end  NameChangeFcn=if exist('rename_tlblock','file')==2,rename_tlblock(gcbh);end  OpenFcn=if exist('tl_open_blockdlg','file')==2,tl_open_blockdlg(gcbh);else,open_system(gcbh,'parameter');end
      mask Help: eval(['if exist(''tl_online_help'',''file'') == 2, tl_online_help(''Topic'',''TL_LogicalOperator''),else, web([''jar:file:///'',matlabroot,''/help/toolbox/simulink/help.jar!/slref/' lower(get_param(gcbh,'Blocktype')) '.html''], ''-helpbrowser''),end'])
      mask Display: plot([-0.05, 1.05, NaN, -0.05, 1.05],[.01, .01, NaN, .99, .99])
  Memory_U : UnitDelay  Description=|  SampleTime=dT  mask(TL_UnitDelay){data={'logdata',{'plotchannels',[]},'output',{'type','Bool'},'state',{'type','Bool'},'date',734383.73416067124}}
      | Unit Delay block of dSPACE TargetLink.
      | 
      | Output signal is equal to the input signal of the last sample step:
      | 
      |         y(k) = u(k-1).
      | 
      | In the 1st sampling step, the output signal is initialized with 'initial condition':
      | 
      |         y(0) = initial condition
      settings: CopyFcn=if exist('tl_reset_reviewflag') == 2, tl_reset_reviewflag(gcbh); end  DeleteFcn=if exist('delete_tlblock','file')==2,delete_tlblock(gcbh);end  NameChangeFcn=if exist('rename_tlblock','file')==2,rename_tlblock(gcbh);end  OpenFcn=if exist('tl_open_blockdlg','file')==2,tl_open_blockdlg(gcbh);else,open_system(gcbh,'parameter');end
      mask Help: eval(['if exist(''tl_online_help'',''file'') == 2, tl_online_help(''Topic'',''TL_UnitDelay''),else, web([''jar:file:///'',matlabroot,''/help/toolbox/simulink/help.jar!/slref/' lower(get_param(gcbh,'Blocktype')) '.html''], ''-helpbrowser''),end'])
      mask Display: plot([-0.05, 1.05, NaN, -0.05, 1.05],[.01, .01, NaN, .99, .99])
  Switch_R : Switch  Description=|  Threshold=1  mask(TL_Switch){data={'logdata',{'plotchannels',[]},'output',{'type','Bool'},'date',734383.73415995366}}
      | Switch block of dSPACE TargetLink.
      | 
      | Passes through input 1 if input 2 is greater than or equal to threshold, otherwise, passes through input 3:
      | 
      | if u2 >= threshold
      |    y = u1;
      | else
      |    y = u3;
      | end
      settings: CopyFcn=if exist('tl_reset_reviewflag') == 2, tl_reset_reviewflag(gcbh); end  DeleteFcn=if exist('delete_tlblock','file')==2,delete_tlblock(gcbh);end  NameChangeFcn=if exist('rename_tlblock','file')==2,rename_tlblock(gcbh);end  OpenFcn=if exist('tl_open_blockdlg','file')==2,tl_open_blockdlg(gcbh);else,open_system(gcbh,'parameter');end
      mask Help: eval(['if exist(''tl_online_help'',''file'') == 2, tl_online_help(''Topic'',''TL_Switch''),else, web([''jar:file:///'',matlabroot,''/help/toolbox/simulink/help.jar!/slref/' lower(get_param(gcbh,'Blocktype')) '.html''], ''-helpbrowser''),end'])
      mask Display: plot([-0.05, 1.05, NaN, -0.05, 1.05],[.01, .01, NaN, .99, .99])
  y : Outport  InitialOutput=0
  wires:
  IV/1 -> Switch_R/1
  Memory_U/1 -> Switch_R/3
  R/1 -> Switch_R/2
  Switch_R/1 -> LogOp_N/1
  u/1 -> Memory_U/1, LogOp_A/1
  LogOp_A/1 -> y/1
  LogOp_N/1 -> LogOp_A/2

== system DAS/DEMO_FAS/DEMO_FAS/Subsystem/DEMO_FAS/DEMO_FAS_Funktion/Tempomat/Tempomat_Function/CC_SetValue/False ==
  Zero : Constant  Description=|  Value=0  SampleTime=-1  mask(TL_Constant){data={'output',{'tolerance',0},'date',734383.73403155094}}
      | Constant block of dSPACE TargetLink.
      | 
      | Output signal keeps the given constant value.
      settings: DeleteFcn=if exist('delete_tlblock','file')==2,delete_tlblock(gcbh);end  NameChangeFcn=if exist('rename_tlblock','file')==2,rename_tlblock(gcbh);end  OpenFcn=if exist('tl_open_blockdlg','file')==2,tl_open_blockdlg(gcbh);else,open_system(gcbh,'parameter');end
      mask Help: eval(['if exist(''tl_online_help'',''file'') == 2, tl_online_help(''Topic'',''TL_Constant''),else, web([''jar:file:///'',matlabroot,''/help/toolbox/simulink/help.jar!/slref/' lower(get_param(gcbh,'Blocktype')) '.html''], ''-helpbrowser''),end'])
      mask Display: plot([-0.05, 1.05, NaN, -0.05, 1.05],[.01, .01, NaN, .99, .99])
  y : Outport
  wires:
  Zero/1 -> y/1

== system DAS/DEMO_FAS/DEMO_FAS/Subsystem/DEMO_FAS/DEMO_FAS_Funktion/Tempomat/Tempomat_Function/CC_SetValue/RSFlipFlop ==
  S : Inport
  R : Inport  Port=2
  LogOp_N : Logic  Description=|  Operator=NOT  Inputs=1  AllPortsSameDT=off  mask(TL_LogicalOperator){data={'logdata',{'plotchannels',[]},'date',734383.73415922455}}
      | Logical operator block of dSPACE TargetLink.
      | 
      | The Logical Operator block performs any of these logical operations on its inputs: AND, OR, NAND, NOR, XOR, and NOT. A nonzero input is treated as TRUE (1), a zero input as FALSE (0). The output depends on the selected operator. The output is 1 if TRUE and 0 if FALSE.
      settings: DeleteFcn=if exist('delete_tlblock','file')==2,delete_tlblock(gcbh);end  NameChangeFcn=if exist('rename_tlblock','file')==2,rename_tlblock(gcbh);end  OpenFcn=if exist('tl_open_blockdlg','file')==2,tl_open_blockdlg(gcbh);else,open_system(gcbh,'parameter');end
      mask Help: eval(['if exist(''tl_online_help'',''file'') == 2, tl_online_help(''Topic'',''TL_LogicalOperator''),else, web([''jar:file:///'',matlabroot,''/help/toolbox/simulink/help.jar!/slref/' lower(get_param(gcbh,'Blocktype')) '.html''], ''-helpbrowser''),end'])
      mask Display: plot([-0.05, 1.05, NaN, -0.05, 1.05],[.01, .01, NaN, .99, .99])
  Memory_Q : UnitDelay  Description=|  SampleTime=dT  mask(TL_UnitDelay){data={'logdata',{'plotchannels',[]},'output',{'type','Bool'},'state',{'type','Bool'},'date',734383.73415886576}}
      | Unit Delay block of dSPACE TargetLink.
      | 
      | Output signal is equal to the input signal of the last sample step:
      | 
      |         y(k) = u(k-1).
      | 
      | In the 1st sampling step, the output signal is initialized with 'initial condition':
      | 
      |         y(0) = initial condition
      settings: CopyFcn=if exist('tl_reset_reviewflag') == 2, tl_reset_reviewflag(gcbh); end  DeleteFcn=if exist('delete_tlblock','file')==2,delete_tlblock(gcbh);end  NameChangeFcn=if exist('rename_tlblock','file')==2,rename_tlblock(gcbh);end  OpenFcn=if exist('tl_open_blockdlg','file')==2,tl_open_blockdlg(gcbh);else,open_system(gcbh,'parameter');end
      mask Help: eval(['if exist(''tl_online_help'',''file'') == 2, tl_online_help(''Topic'',''TL_UnitDelay''),else, web([''jar:file:///'',matlabroot,''/help/toolbox/simulink/help.jar!/slref/' lower(get_param(gcbh,'Blocktype')) '.html''], ''-helpbrowser''),end'])
      mask Display: plot([-0.05, 1.05, NaN, -0.05, 1.05],[.01, .01, NaN, .99, .99])
  One_S : Constant  Description=|  mask(TL_Constant){data={'date',734383.73415796296}}
      | Constant block of dSPACE TargetLink.
      | 
      | Output signal keeps the given constant value.
      settings: DeleteFcn=if exist('delete_tlblock','file')==2,delete_tlblock(gcbh);end  NameChangeFcn=if exist('rename_tlblock','file')==2,rename_tlblock(gcbh);end  OpenFcn=if exist('tl_open_blockdlg','file')==2,tl_open_blockdlg(gcbh);else,open_system(gcbh,'parameter');end
      mask Help: eval(['if exist(''tl_online_help'',''file'') == 2, tl_online_help(''Topic'',''TL_Constant''),else, web([''jar:file:///'',matlabroot,''/help/toolbox/simulink/help.jar!/slref/' lower(get_param(gcbh,'Blocktype')) '.html''], ''-helpbrowser''),end'])
      mask Display: plot([-0.05, 1.05, NaN, -0.05, 1.05],[.01, .01, NaN, .99, .99])
  Switch_R : Switch  Description=|  Threshold=1  mask(TL_Switch){data={'logdata',{'plotchannels',[]},'output',{'type','Bool'},'date',734383.73415760417}}
      | Switch block of dSPACE TargetLink.
      | 
      | Passes through input 1 if input 2 is greater than or equal to threshold, otherwise, passes through input 3:
      | 
      | if u2 >= threshold
      |    y = u1;
      | else
      |    y = u3;
      | end
      settings: CopyFcn=if exist('tl_reset_reviewflag') == 2, tl_reset_reviewflag(gcbh); end  DeleteFcn=if exist('delete_tlblock','file')==2,delete_tlblock(gcbh);end  NameChangeFcn=if exist('rename_tlblock','file')==2,rename_tlblock(gcbh);end  OpenFcn=if exist('tl_open_blockdlg','file')==2,tl_open_blockdlg(gcbh);else,open_system(gcbh,'parameter');end
      mask Help: eval(['if exist(''tl_online_help'',''file'') == 2, tl_online_help(''Topic'',''TL_Switch''),else, web([''jar:file:///'',matlabroot,''/help/toolbox/simulink/help.jar!/slref/' lower(get_param(gcbh,'Blocktype')) '.html''], ''-helpbrowser''),end'])
      mask Display: plot([-0.05, 1.05, NaN, -0.05, 1.05],[.01, .01, NaN, .99, .99])
  Switch_S : Switch  Description=|  Threshold=1  mask(TL_Switch){data={'logdata',{'plotchannels',[]},'output',{'type','Bool'},'date',734383.73415668984}}
      | Switch block of dSPACE TargetLink.
      | 
      | Passes through input 1 if input 2 is greater than or equal to threshold, otherwise, passes through input 3:
      | 
      | if u2 >= threshold
      |    y = u1;
      | else
      |    y = u3;
      | end
      settings: CopyFcn=if exist('tl_reset_reviewflag') == 2, tl_reset_reviewflag(gcbh); end  DeleteFcn=if exist('delete_tlblock','file')==2,delete_tlblock(gcbh);end  NameChangeFcn=if exist('rename_tlblock','file')==2,rename_tlblock(gcbh);end  OpenFcn=if exist('tl_open_blockdlg','file')==2,tl_open_blockdlg(gcbh);else,open_system(gcbh,'parameter');end
      mask Help: eval(['if exist(''tl_online_help'',''file'') == 2, tl_online_help(''Topic'',''TL_Switch''),else, web([''jar:file:///'',matlabroot,''/help/toolbox/simulink/help.jar!/slref/' lower(get_param(gcbh,'Blocktype')) '.html''], ''-helpbrowser''),end'])
      mask Display: plot([-0.05, 1.05, NaN, -0.05, 1.05],[.01, .01, NaN, .99, .99])
  Zero_R : Constant  Description=|  Value=0  mask(TL_Constant){data={'date',734383.73415597226}}
      | Constant block of dSPACE TargetLink.
      | 
      | Output signal keeps the given constant value.
      settings: DeleteFcn=if exist('delete_tlblock','file')==2,delete_tlblock(gcbh);end  NameChangeFcn=if exist('rename_tlblock','file')==2,rename_tlblock(gcbh);end  OpenFcn=if exist('tl_open_blockdlg','file')==2,tl_open_blockdlg(gcbh);else,open_system(gcbh,'parameter');end
      mask Help: eval(['if exist(''tl_online_help'',''file'') == 2, tl_online_help(''Topic'',''TL_Constant''),else, web([''jar:file:///'',matlabroot,''/help/toolbox/simulink/help.jar!/slref/' lower(get_param(gcbh,'Blocktype')) '.html''], ''-helpbrowser''),end'])
      mask Display: plot([-0.05, 1.05, NaN, -0.05, 1.05],[.01, .01, NaN, .99, .99])
  Q : Outport  InitialOutput=0
  NOT_Q : Outport  Port=2  InitialOutput=0
  wires:
  LogOp_N/1 -> NOT_Q/1
  R/1 -> Switch_R/2
  Zero_R/1 -> Switch_R/1
  Switch_R/1 -> LogOp_N/1, Q/1, Memory_Q/1
  S/1 -> Switch_S/2
  One_S/1 -> Switch_S/1
  Switch_S/1 -> Switch_R/3
  Memory_Q/1 -> Switch_S/3
